simulink model "UPS_3level_Ttype_Inverter_simplified_ctrl"  (R2012b)
settings: Solver=ode4  StartTime=0.0  StopTime=Tfinal  FixedStep=Ts  MaxStep=1e-5  RelTol=1e-3
values from neighbouring files (symbols this model uses):
  Ts = 1/(1*1e6)    (= 1e-06)    [Run.m]
  Vd = 720    [Run.m]
  VSI = rmfield(VSI, {'IF1', 'IF2', 'FLUXlin1', 'FLUXlin2',      'FLUXnonlin1', 'FLUXnonlin2', 'Lfnonlin'})    [Run.m]
undefined symbols (not defined in the file or in its folder): ADC, CTRL, DiscIntNeverNeededParam, PR, S, UPS
libraries: powerlib x113, simulink_extras x11, powerlib_extras x11, simulink x3
(part 3 of 3)

== system UPS_3level_Ttype_Inverter_simplified_ctrl/Output Inverter Control System SRF(dq0) - SPWM /SPWM (Treg)2/controller ph a1/vCf reference ==
  cos* sin* : Inport
  vs* [V] : Inport  Port=2
  Product3 : Product  RndMeth=Zero
  vCf_ref [V] : Outport
  wires:
  vs* [V]/1 -> Product3/2
  Product3/1 -> vCf_ref [V]/1
  cos* sin*/1 -> Product3/1

== system UPS_3level_Ttype_Inverter_simplified_ctrl/Output Inverter Control System SRF(dq0) - SPWM /SPWM (Treg)2/controller ph a2/Kalman Estimation fundamental ==
  iLoad [A] : Inport
  Demux2 : Demux  Outputs=2
  Discrete State-Space4 : DiscreteStateSpace  A=CTRL.AKd2  B=CTRL.BKd2  C=CTRL.CKd2  D=CTRL.DKd2  X0=[0;0]  SampleTime=-1
  iLoad_est cos [A] : Outport
  iLoad_est sin [A] : Outport  Port=2
  wires:
  Demux2/2 -> iLoad_est sin [A]/1
  Demux2/1 -> iLoad_est cos [A]/1
  Discrete State-Space4/1 -> Demux2/1
  iLoad [A]/1 -> Discrete State-Space4/1

== system UPS_3level_Ttype_Inverter_simplified_ctrl/Output Inverter Control System SRF(dq0) - SPWM /SPWM (Treg)2/controller ph a2/LQR gain ==
  iLf error [A] : Inport
  vCf error [V] : Inport  Port=2
  Add3 : Sum
  Gain : Gain  Gain=CTRL.Klq(1)
  Gain3 : Gain  Gain=CTRL.Klq(2)
  delta u [V] : Outport
  wires:
  Add3/1 -> delta u [V]/1
  iLf error [A]/1 -> Gain/1
  vCf error [V]/1 -> Gain3/1
  Gain/1 -> Add3/1
  Gain3/1 -> Add3/2

== system UPS_3level_Ttype_Inverter_simplified_ctrl/Output Inverter Control System SRF(dq0) - SPWM /SPWM (Treg)2/controller ph a2/vCf reference ==
  cos* sin* : Inport
  vs* [V] : Inport  Port=2
  Product3 : Product  RndMeth=Zero
  vCf_ref [V] : Outport
  wires:
  cos* sin*/1 -> Product3/1
  Product3/1 -> vCf_ref [V]/1
  vs* [V]/1 -> Product3/2

== system UPS_3level_Ttype_Inverter_simplified_ctrl/Output Inverter Control System SRF(dq0) - SPWM /SPWM (Treg)2/controller ph a3/Kalman Estimation fundamental ==
  iLoad [A] : Inport
  Demux2 : Demux  Outputs=2
  Discrete State-Space4 : DiscreteStateSpace  A=CTRL.AKd2  B=CTRL.BKd2  C=CTRL.CKd2  D=CTRL.DKd2  X0=[0;0]  SampleTime=-1
  iLoad_est cos [A] : Outport
  iLoad_est sin [A] : Outport  Port=2
  wires:
  iLoad [A]/1 -> Discrete State-Space4/1
  Discrete State-Space4/1 -> Demux2/1
  Demux2/1 -> iLoad_est cos [A]/1
  Demux2/2 -> iLoad_est sin [A]/1

== system UPS_3level_Ttype_Inverter_simplified_ctrl/Output Inverter Control System SRF(dq0) - SPWM /SPWM (Treg)2/controller ph a3/LQR gain ==
  iLf error [A] : Inport
  vCf error [V] : Inport  Port=2
  Add3 : Sum
  Gain : Gain  Gain=CTRL.Klq(1)
  Gain3 : Gain  Gain=CTRL.Klq(2)
  delta u [V] : Outport
  wires:
  Gain3/1 -> Add3/2
  Gain/1 -> Add3/1
  vCf error [V]/1 -> Gain3/1
  iLf error [A]/1 -> Gain/1
  Add3/1 -> delta u [V]/1

== system UPS_3level_Ttype_Inverter_simplified_ctrl/Output Inverter Control System SRF(dq0) - SPWM /SPWM (Treg)2/controller ph a3/vCf reference ==
  cos* sin* : Inport
  vs* [V] : Inport  Port=2
  Product3 : Product  RndMeth=Zero
  vCf_ref [V] : Outport
  wires:
  vs* [V]/1 -> Product3/2
  Product3/1 -> vCf_ref [V]/1
  cos* sin*/1 -> Product3/1
